simulink model "CLIK_SCND"  (R2023a)
settings: Solver=ode1  StartTime=0.0  StopTime=25  FixedStep=Ts  RelTol=1e-3
values from neighbouring files (symbols this model uses):
  Ts = 0.001    [TRAJ.m]
undefined symbols (not defined in the file or in its folder): DiscIntNeverNeededParam
settings Model: Creator=39388  LastModifiedBy=39388

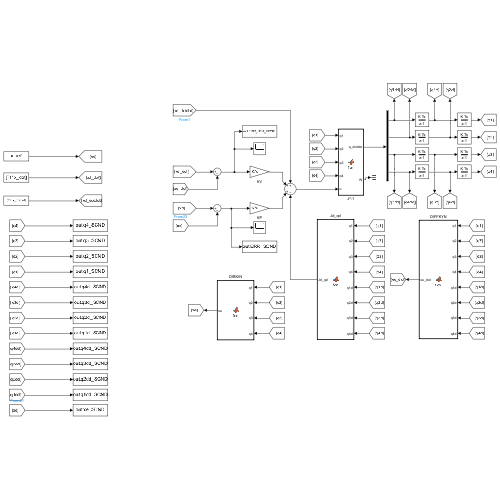
[thumbnail: Simulink's stored preview of the top-level diagram]
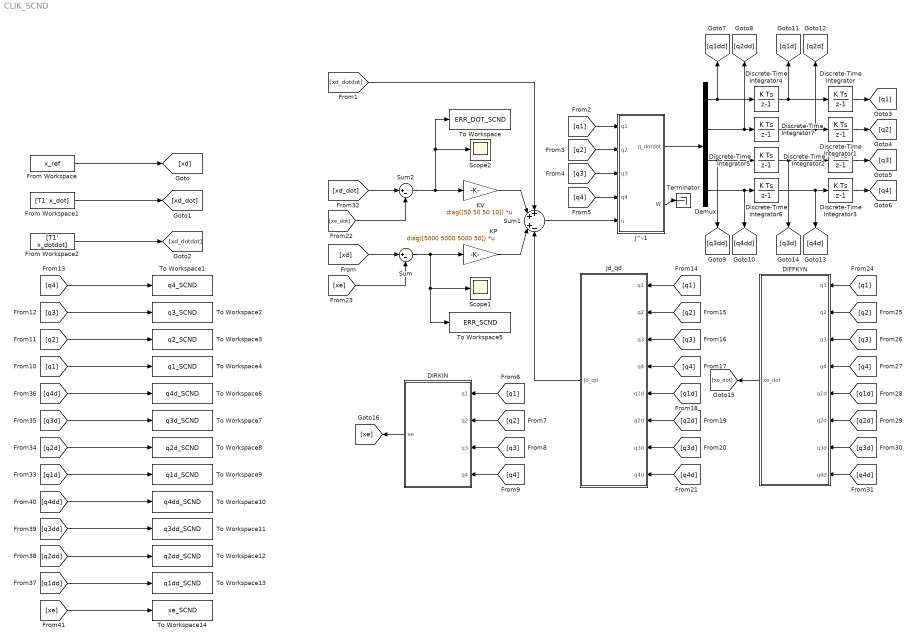
== system CLIK_SCND ==
  DIFFKYN : MATLAB Function  TreatAsAtomicUnit=on
  DIRKIN : MATLAB Function  TreatAsAtomicUnit=on
  Demux : Demux
  Discrete-Time Integrator{,4..7} (5 alike) : DiscreteIntegrator  SampleTime=Ts  ICPrevOutput=DiscIntNeverNeededParam  ICPrevScaledInput=DiscIntNeverNeededParam
  Discrete-Time Integrator1 : DiscreteIntegrator  InitialCondition=pi/2  SampleTime=Ts  ICPrevOutput=DiscIntNeverNeededParam  ICPrevScaledInput=DiscIntNeverNeededParam
  Discrete-Time Integrator2 : DiscreteIntegrator  InitialCondition=-0.25  SampleTime=Ts  ICPrevOutput=DiscIntNeverNeededParam  ICPrevScaledInput=DiscIntNeverNeededParam
  Discrete-Time Integrator3 : DiscreteIntegrator  InitialCondition=-pi  SampleTime=Ts  ICPrevOutput=DiscIntNeverNeededParam  ICPrevScaledInput=DiscIntNeverNeededParam
  From Workspace : FromWorkspace  VariableName=x_ref
  From Workspace1 : FromWorkspace  VariableName=[T1' x_dot]
  From Workspace2 : FromWorkspace  VariableName=[T1' x_dotdot]
  J^-1 : MATLAB Function  TreatAsAtomicUnit=on
  Jd_qd : MATLAB Function  TreatAsAtomicUnit=on
  KP : Gain  Gain=diag([5000 5000 5000 50])  Multiplication=Matrix(K*u)
  KV : Gain  Gain=diag([50 50 50 10])  Multiplication=Matrix(K*u)
  Scope1 : Scope
  Scope2 : Scope
  Sum : Sum  Inputs=|+-
  Sum1 : Sum  Inputs=++|+-
  Sum2 : Sum  Inputs=|+-
  Terminator : Terminator
  To Workspace : ToWorkspace  VariableName=ERR_DOT_SCND  SaveFormat=Structure With Time  SampleTime=-1
  To Workspace1 : ToWorkspace  VariableName=q4_SCND  SaveFormat=Structure With Time  SampleTime=-1
  To Workspace10 : ToWorkspace  VariableName=q4dd_SCND  SaveFormat=Structure With Time  SampleTime=-1
  To Workspace11 : ToWorkspace  VariableName=q3dd_SCND  SaveFormat=Structure With Time  SampleTime=-1
  To Workspace12 : ToWorkspace  VariableName=q2dd_SCND  SaveFormat=Structure With Time  SampleTime=-1
  To Workspace13 : ToWorkspace  VariableName=q1dd_SCND  SaveFormat=Structure With Time  SampleTime=-1
  To Workspace14 : ToWorkspace  VariableName=xe_SCND  SaveFormat=Structure With Time  SampleTime=-1
  To Workspace2 : ToWorkspace  VariableName=q3_SCND  SaveFormat=Structure With Time  SampleTime=-1
  To Workspace3 : ToWorkspace  VariableName=q2_SCND  SaveFormat=Structure With Time  SampleTime=-1
  To Workspace4 : ToWorkspace  VariableName=q1_SCND  SaveFormat=Structure With Time  SampleTime=-1
  To Workspace5 : ToWorkspace  VariableName=ERR_SCND  SaveFormat=Structure With Time  SampleTime=-1
  To Workspace6 : ToWorkspace  VariableName=q4d_SCND  SaveFormat=Structure With Time  SampleTime=-1
  To Workspace7 : ToWorkspace  VariableName=q3d_SCND  SaveFormat=Structure With Time  SampleTime=-1
  To Workspace8 : ToWorkspace  VariableName=q2d_SCND  SaveFormat=Structure With Time  SampleTime=-1
  To Workspace9 : ToWorkspace  VariableName=q1d_SCND  SaveFormat=Structure With Time  SampleTime=-1
  wires:
  From Workspace1/1 -> [xd_dot]
  From Workspace2/1 -> [xd_dotdot]
  [xd] -> Sum/1
  Sum/1 -> To Workspace5/1, Scope1/1, KP/1
  Sum1/1 -> J^-1/5(u)
  [xd_dotdot] -> Sum1/1
  From Workspace/1 -> [xd]
  J^-1/1(q_dotdot) -> Demux/1
  [q1] -> J^-1/1(q1)
  [q2] -> J^-1/2(q2)
  [q3] -> J^-1/3(q3)
  [q4] -> J^-1/4(q4)
  [q1] -> DIRKIN/1(q1)
  [q2] -> DIRKIN/2(q2)
  [q3] -> DIRKIN/3(q3)
  [q4] -> DIRKIN/4(q4)
  J^-1/2(W) -> Terminator/1
  [q4] -> To Workspace1/1
  [q3] -> To Workspace2/1
  [q2] -> To Workspace3/1
  [q1] -> To Workspace4/1
  Discrete-Time Integrator/1 -> [q1]
  Discrete-Time Integrator1/1 -> [q2]
  Discrete-Time Integrator2/1 -> [q3]
  Discrete-Time Integrator3/1 -> [q4]
  Discrete-Time Integrator4/1 -> [q1d], Discrete-Time Integrator/1
  Demux/1 -> Discrete-Time Integrator4/1, [q1dd]
  Discrete-Time Integrator7/1 -> [q2d], Discrete-Time Integrator1/1
  Demux/2 -> [q2dd], Discrete-Time Integrator7/1
  Discrete-Time Integrator5/1 -> [q3d], Discrete-Time Integrator2/1
  Demux/3 -> [q3dd], Discrete-Time Integrator5/1
  Discrete-Time Integrator6/1 -> [q4d], Discrete-Time Integrator3/1
  Demux/4 -> [q4dd], Discrete-Time Integrator6/1
  KP/1 -> Sum1/3
  [q1] -> Jd_qd/1(q1)
  [q2] -> Jd_qd/2(q2)
  [q3] -> Jd_qd/3(q3)
  [q4] -> Jd_qd/4(q4)
  [q1d] -> Jd_qd/5(q1d)
  [q2d] -> Jd_qd/6(q2d)
  [q3d] -> Jd_qd/7(q3d)
  [q4d] -> Jd_qd/8(q4d)
  Jd_qd/1(Jd_qd) -> Sum1/4
  DIFFKYN/1(xe_dot) -> [xe_dot]
  DIRKIN/1(xe) -> [xe]
  [xe] -> Sum/2
  [q1] -> DIFFKYN/1(q1)
  [q2] -> DIFFKYN/2(q2)
  [q3] -> DIFFKYN/3(q3)
  [q4] -> DIFFKYN/4(q4)
  [q1d] -> DIFFKYN/5(q1d)
  [q2d] -> DIFFKYN/6(q2d)
  [q3d] -> DIFFKYN/7(q3d)
  [q4d] -> DIFFKYN/8(q4d)
  [xd_dot] -> Sum2/1
  [xe_dot] -> Sum2/2
  Sum2/1 -> To Workspace/1, Scope2/1, KV/1
  KV/1 -> Sum1/2
  [q4d] -> To Workspace6/1
  [q3d] -> To Workspace7/1
  [q2d] -> To Workspace8/1
  [q1d] -> To Workspace9/1
  [q2dd] -> To Workspace12/1
  [q3dd] -> To Workspace11/1
  [q4dd] -> To Workspace10/1
  [q1dd] -> To Workspace13/1
  [xe] -> To Workspace14/1

== matlab function CLIK_SCND/DIRKIN ==
  data: q1 input; xe output; q2 input; q3 input; q4 input
function xe = fcn(q1,q2,q3,q4)

xe=[0.5*cos(q1)+0.5*cos(q1+q2);
    0.5*sin(q1)+0.5*sin(q1+q2);
    1+q3;
    q1+q2+q4];

== matlab function CLIK_SCND/J^-1 ==
  data: q1 input; q2 input; q3 input; q4 input; u input; q_dotdot output; W output
function  [q_dotdot,W] = fcn(q1,q2,q3,q4,u)

    J=[-0.5*sin(q1-0.5*sin(q1+q2)) -0.5*sin(q1+q2) 0 0;
        0.5*cos(q1-0.5*cos(q1+q2))  0.5*cos(q1+q2) 0 0;
        0                               0                 1 0;
        1                               1                 0 1];

     q_dotdot=J\u;
     
     W=0.5^2*abs(sin(q2));

== matlab function CLIK_SCND/Jd_qd ==
  data: q1 input; Jd_qd output; q2 input; q3 input; q4 input; q1d input; q2d input; q3d input; q4d input
function Jd_qd = fcn(q1,q2,q3,q4,q1d,q2d,q3d,q4d)

J_dot=[-0.5*q1d*cos(q1)-0.5*(q1d+q2d)*cos(q1+q2) -0.5*(q1d+q2d)*cos(q1+q2) 0 0;
       -0.5*q1d*sin(q1)-0.5*(q1d+q2d)*sin(q1+q2) -0.5*(q1d+q2d)*sin(q1+q2) 0 0;
        0                                         0                        0 0;
        0                                         0                        0 0];

Jd_qd=J_dot*[q1d; q2d; q3d; q4d];

== matlab function CLIK_SCND/DIFFKYN ==
  data: q1 input; xe_dot output; q2 input; q3 input; q4 input; q1d input; q2d input; q3d input; q4d input
function xe_dot = fcn(q1,q2,q3,q4,q1d,q2d,q3d,q4d)

J=[-0.5*sin(q1-0.5*sin(q1+q2)) -0.5*sin(q1+q2) 0 0;
    0.5*cos(q1-0.5*cos(q1+q2))  0.5*cos(q1+q2) 0 0;
    0                           0              1 0;
    1                           1              0 1];

xe_dot=J*[q1d;q2d;q3d;q4d];
